simulink model "SR_SNN_Extrinsic_code"  (R2022a)
settings: Solver=FixedStepAuto  StartTime=0.0  StopTime=NTimeSteps  FixedStep=Ts  RelTol=1e-3
values from neighbouring files (symbols this model uses):
  a1 = 5    [SR_Main_Script_Sim.m]
  b = 2    [SR_Main_Script_Sim.m]
  Etol = 10    [SR_Main_Script_Sim.m]
  Mu = 0    [SR_Main_Script_Sim.m]
  NObservations = 10    [SR_Main_Script_Sim.m]
  NStepPerTarget = NTimeSteps/NObservations    (= 1)    [SR_Main_Script_Sim.m]
  r = 0.14*0.5*10    (= 0.7)    [SR_Main_Script_Sim.m]
  s1 = 900    [ConditionCheck.m]    (also in MySNN.m = 0)
  s2 = 900    [ConditionCheck.m]    (also in MySNN.m = 0)
  s3 = 900    [ConditionCheck.m]    (also in MySNN.m = 0)
  Ts = 1e-3    (= 0.001)    [SR_Main_Script_Sim.m]
  Tx = 1    [SR_Main_Script_Sim.m]
  Txi = r*cos(xx)    [SR_Main_Script_Sim.m]
  Ty = 1    [SR_Main_Script_Sim.m]
  Tyi = r*sin(xx)    [SR_Main_Script_Sim.m]
  Tz = 2    [SR_Main_Script_Sim.m]
  v1 = v1 - vMax*(s3/sMin)    [ConditionCheck.m]
  v2 = v2 - vMax*(s3/sMin)    [ConditionCheck.m]
  v3 = v3 - vMax*(s2/sMin)    [ConditionCheck.m]
  v4 = 0    [ConditionCheck.m]
  v5 = 0    [ConditionCheck.m]
  v6 = 0    [ConditionCheck.m]
  v7 = 0    [ConditionCheck.m]
  v8 = 0    [ConditionCheck.m]
  Var = 5    [SR_Main_Script_Sim.m]
  x_i = [[1] ... (first row only)    [SR_Main_Script_Sim.m]
undefined symbols (not defined in the file or in its folder): ConditionCheck, dev_handle, s4, s5, s6, setSup, U1, U2, U3
libraries: slpidlib x4, cstblocks x3
settings Model: SimulationMode=accelerator  Creator=Pouya  LastModifiedBy=Pouya
settings DebuggingCC: UnconnectedInputMsg=warning  UnconnectedOutputMsg=warning  UnconnectedLineMsg=warning
settings RTWCC: DLArmComputeVersion=19.05

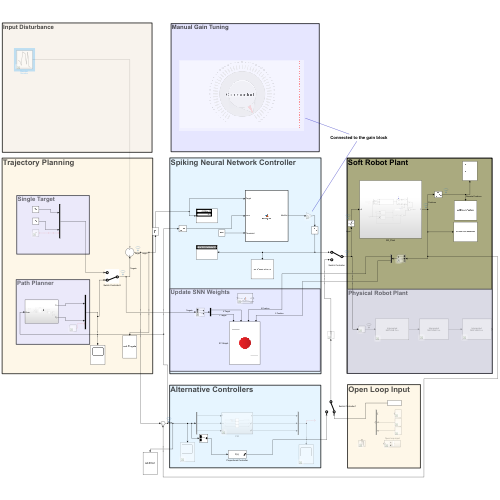
[thumbnail: Simulink's stored preview of the top-level diagram]
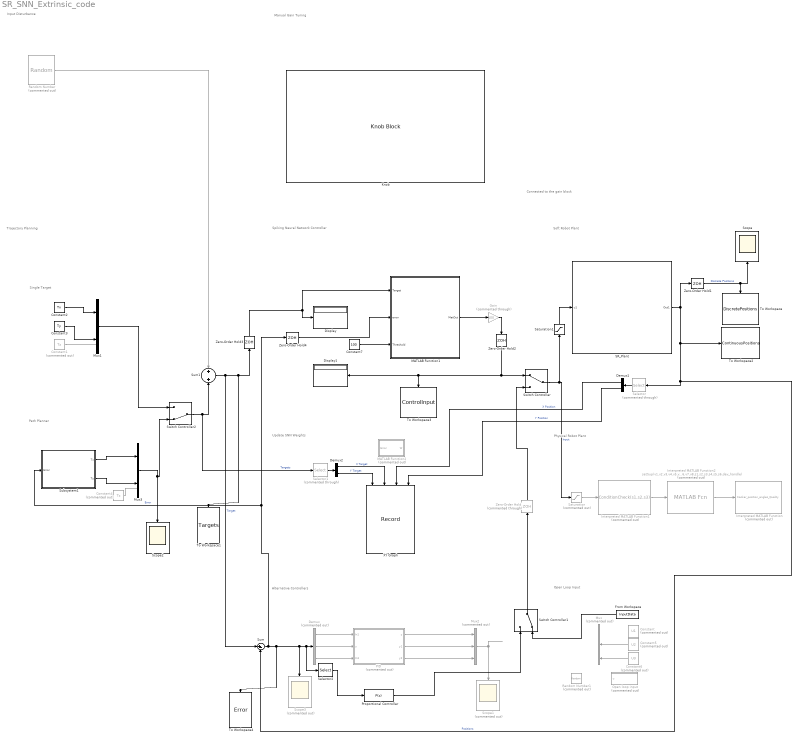
== system SR_SNN_Extrinsic_code ==
  note: Connected to the gain block
  note: Manual Gain Tuning
  note: Physical Robot Plant
  note: Update SNN Weights
  note: Input Disturbance
  note: Path Planner
  note: Single Target
  note: Open Loop Input
  note: Alternative Controllers
  note: Trajectory Planning
  note: Soft Robot Plant
  note: Spiking Neural Network Controller
  Constant : Constant  Commented=on  Value=U1
  Constant1 : Constant  Commented=on  Value=Tz
  Constant2 : Constant  Value=Tx
  Constant3 : Constant  Value=Ty
  Constant4 : Constant  Commented=on  Value=Tz
  Constant5 : Constant  Commented=on  Value=U2
  Constant6 : Constant  Commented=on  Value=U3
  Constant7 : Constant  Value=100
  Demux : Demux  Commented=on  Outputs=3
  Demux1 : Demux  Outputs=2
  Demux2 : Demux  Outputs=2
  Display : Display
  Display1 : Display
  From Workspace : FromWorkspace  VariableName=InputData  SampleTime=Ts
  Gain : Gain  Commented=through  Gain=100
  Interpreted MATLAB Function : MATLABFcn  Commented=on  MATLABFcn=tracker_position_angles_Quality
  Interpreted MATLAB Function1 : MATLABFcn  Commented=on  MATLABFcn=ConditionCheck(s1,s2,s3)
  Interpreted MATLAB Function2 : MATLABFcn  Commented=on  MATLABFcn=setSup(v1,v2,v3,v4,v5,v6,v7,v8,s1,s2,s3,s4,s5,s6,dev_handle)
  Knob : KnobBlock
  MATLAB Function1 : MATLAB Function  TreatAsAtomicUnit=on
  MATLAB Function2 : MATLAB Function  Commented=on  TreatAsAtomicUnit=on
  Mux : Mux  Commented=on  Inputs=3
  Mux1 : Mux  Inputs=2
  Mux2 : Mux  Commented=on  Inputs=3
  Mux3 : Mux  Inputs=2
  Open loop input : Subsystem  Commented=on
  PID : Subsystem  Commented=on
  Proportional Controller : slpidlib/PID Controller  Controller=P  Form=Parallel  TimeDomain=Discrete-time  UseExternalTs=off  SampleTime=-1  IntegratorMethod=Forward Euler  FilterMethod=Forward Euler  ControllerParametersSource=internal  P=150  I=0.1  UseKiTs=off  D=0  N=100  UseFilter=on  TunerSelectOption=Transfer Function Based (PID Tuner App)  InitialConditionSource=internal  InitialConditionForIntegrator=1  InitialConditionForFilter=0  DifferentiatorICPrevScaledInput=0  ExternalReset=none  TrackingMode=off  Kt=1  LimitOutput=on  SatLimitsSource=internal  UpperSaturationLimit=1  LowerSaturationLimit=0  LinearizeAsGain=off  AntiWindupMode=none  Kb=1  POutMin=[]  POutMax=[]  IOutMin=[]  IOutMax=[]  DOutMin=[]  DOutMax=[]  NOutMin=[]  NOutMax=[]  SumOutMin=[]  SumOutMax=[]  SaturationOutMin=[]  SaturationOutMax=[]  PParamMin=[]  PParamMax=[]  IParamMin=[]  IParamMax=[]  DParamMin=[]  DParamMax=[]  NParamMin=[]  NParamMax=[]  KbParamMin=[]  KbParamMax=[]  KtParamMin=[]  KtParamMax=[]  KbOutMin=[]  KbOutMax=[]  KtOutMin=[]  KtOutMax=[]  IntegratorOutMin=[]  IntegratorOutMax=[]  FilterOutMin=[]  FilterOutMax=[]  SumI1OutMin=[]  SumI1OutMax=[]  SumI2OutMin=[]  SumI2OutMax=[]  SumI3OutMin=[]  SumI3OutMax=[]  SumI4OutMin=[]  SumI4OutMax=[]  SumDOutMin=[]  SumDOutMax=[]  DifferentiatorOutMin=[]  DifferentiatorOutMax=[]  FilterDiffOutCoefMin=[]  FilterDiffOutCoefMax=[]  ReciprocalOutMin=[]  ReciprocalOutMax=[]  SumDenOutMin=[]  SumDenOutMax=[]  SumNumOutMin=[]  SumNumOutMax=[]  DivideOutMin=[]  DivideOutMax=[]  UdiffTsProdOutMin=[]  UdiffTsProdOutMax=[]  NTsProdOutMin=[]  NTsProdOutMax=[]  UintegralTsProdOutMin=[]  UintegralTsProdOutMax=[]  UngainTsProdOutMin=[]  UngainTsProdOutMax=[]  IntegratorContinuousStateAttributes=''  IntegratorStateMustResolveToSignalObject=off  IntegratorRTWStateStorageClass=Auto  FilterContinuousStateAttributes=''  FilterStateMustResolveToSignalObject=off  FilterRTWStateStorageClass=Auto  ParallelPVariant=InternalParameters  IdealPVariant=Disabled  IVariant=Disabled  DVariant=Disabled  IntegratorVariant=Disabled  SatVariant=Enabled  AWVariant=Disabled  PCopyVariant=Disabled  TRVariant=Disabled  FdbkBlocksVariant=Forward  IdealPFdbkVariant=Disabled  SatFdbkVariant=Disabled  DerivativeFilterVariant=Disabled  NVariant=Disabled  NCopyVariant=Disabled_SignalSpec  FilterICVariant=Disabled  IntegratorICVariant=Disabled  ExternalResetVariant=Disabled  TRSumVariant=Passthrough  SumFdbkVariant=Disabled  SumVariant=Passthrough_P  TsampFilterVariant=InternalTs  TsampNgainVariant=Passthrough  TsampIntegralVariant=Disabled_SignalSpec  ExternalSaturationOutDataTypeStr=Inherit: Same as second input  aMode=0
  Random Number : RandomNumber  Commented=on  Mean=Mu  Variance=Var  SampleTime=Ts
  Random Number1 : RandomNumber  Commented=on  SampleTime=Ts
  SR_Plant : Subsystem
  Saturation : Saturate  Commented=on  UpperLimit=4  LowerLimit=-4
  Saturation1 : Saturate  UpperLimit=1  LowerLimit=0
  Scope : Scope
  Scope1 : Scope  Commented=on
  Scope2 : Scope
  Scope3 : Scope  Commented=on
  Selector : Selector  Commented=through  InputPortWidth=3  IndexOptions=Index vector (dialog)  Indices=[1 2]  OutputSizes=1
  Selector1 : Selector  Commented=through  InputPortWidth=3  IndexOptions=Index vector (dialog)  Indices=[1 2]  OutputSizes=1
  Selector2 : Selector  InputPortWidth=2  IndexOptions=Index vector (dialog)  Indices=[1]  OutputSizes=1
  Subsystem1 : Subsystem
  Sum : Sum  Inputs=|+-
  Sum1 : Sum
  Switch Controller : ManualSwitch
  Switch Controller1 : ManualSwitch  CurrentSetting=0
  Switch Controller2 : ManualSwitch  CurrentSetting=0
  To Workspace : ToWorkspace  VariableName=DiscretePositions  SaveFormat=Timeseries  SampleTime=-1
  To Workspace1 : ToWorkspace  VariableName=Targets  SaveFormat=Timeseries  SampleTime=-1
  To Workspace2 : ToWorkspace  VariableName=ContinuousPositions  SaveFormat=Timeseries  SampleTime=-1
  To Workspace3 : ToWorkspace  VariableName=ControlInput  SaveFormat=Timeseries  SampleTime=-1
  To Workspace4 : ToWorkspace  VariableName=Error  SaveFormat=Timeseries  SampleTime=-1
  XY Graph : Record  FileSettingsInternal="{\"entries\":[{\"content\":{\"excelSettings\":{\"content\":{},\"type\":\"Streamout.ExcelSettings\"}},\"type\":\"Streamout.FileSettingStorage\",\"uuid\":\"73c5b73b-fab0-4ab5-94d2-4132d8f4e88e\"}],\"packageUris\":[\"http://schema.mathworks.com/mf0/streamout_blocks/R2020a\"],\"version\":\"1.0\"}"  Layout=[1 1]  SignalsInternal="{\"entries\":[{\"content\":{\"signals\":[{\"content\":{\"blockPath\":[\"SR_SNN_Extrinsic_code/XY Graph\"],\"channel\":[],\"dimensions\":[1],\"domain\":\"SR_SNN_Extrinsic_code/XY Graph\",\"lineColor\":\"#0072bd\",\"plots\":[1,2],\"port\":1,\"sid\":[\"\"],\"signalID\":6157,\"signalName\":\"Y Target\"},\"type\":\"RecordBlkView.Signal\",\"uuid\":\"fa4d0461-3b01-48b9-ba2e-6f3d6dd28ef7\"},{\"content\":{\"blockPath\":[\"SR_SNN_Extrinsic_code/XY Graph\"],\"channel\":[],\"dimensions\":[1],\"domain\":\"SR_SNN_Extrinsic_code/XY Graph\",\"lineColor\":\"#0072bd\",\"plots\":[1,2],\"port\":2,\"sid\":[\"\"],\"signalID\":6161,\"signalName\":\"X Target\"},\"type\":\"RecordBlkView.Signal\",\"uuid\":\"838e8c0a-52c2-4c5c-8dac-cd2bc88a20a1\"},{\"content\":{\"blockPath\":[\"SR_SNN_Extrinsic_code/XY Graph\"],\"channel\":[],\"dimensions\":[1],\"domain\":\"SR_SNN_Extrinsic_code/XY Graph\",\"lineColor\":\"#d95319\",\"lineStyle\":\"DOTTED\",\"plots\":[1,2],\"port\":3,\"sid\":[\"\"],\"signalID\":6165,\"signalName\":\"X Position\"},\"type\":\"RecordBlkView.Signal\",\"uuid\":\"8dc49ed9-1307-4fcf-8461-6fcf0d652c4a\"},{\"content\":{\"blockPath\":[\"SR_SNN_Extrinsic_code/XY Graph\"],\"channel\":[],\"dimensions\":[1],\"domain\":\"SR_SNN_Extrinsic_code/XY Graph\",\"lineColor\":\"#d95319\",\"lineStyle\":\"DOTTED\",\"plots\":[1,2],\"port\":4,\"sid\":[\"\"],\"signalID\":6169,\"signalName\":\"Y Position\"},\"type\":\"RecordBlkView.Signal\",\"uuid\":\"e0714d31-97f1-4acd-9cba-ab512efbf2cd\"}]},\"type\":\"RecordBlkView.InputSignals\",\"uuid\":\"e6cc7207-a460-4614-bf63-22bf2ecd2d00\"}],\"packageUris\":[\"http://schema.mathworks.com/mf0/streamout_blocks/R2020a\"],\"version\":\"1.0\"}"  VisualizationBindings="{\"xyplotplugin\":{\"info\":[{\"series\":[{\"bindingParametersList\":[{\"parameter\":\"Y-Axis\",\"signalID\":6157,\"signalName\":\"Y Target\"},{\"parameter\":\"X-Axis\",\"signalID\":6161,\"signalName\":\"X Target\"}],\"seriesID\":9808},{\"bindingParametersList\":[{\"parameter\":\"X-Axis\",\"signalID\":6165,\"signalName\":\"X Position\"},{\"parameter\":\"Y-Axis\",\"signalID\":6169,\"signalName\":\"Y Position\"}],\"seriesID\":48772}],\"subplotID\":1}]}}"  CompatibilityTag=XY
  Zero-Order Hold : ZeroOrderHold  Commented=through  SampleTime=Ts
  Zero-Order Hold{1..4} (4 alike) : ZeroOrderHold  SampleTime=Ts
  wires:
  Constant2/1 -> Mux1/1
  Constant3/1 -> Mux1/2
  SR_Plant/1(Out1) -> Sum/2, Selector/1, To Workspace2/1, Zero-Order Hold1/1  "Positions"
  Constant1/1 -> ?
  Switch Controller1/1 -> Zero-Order Hold/1
  Zero-Order Hold/1 -> Switch Controller/2
  Demux/2 -> PID/2(u)
  Demux/1 -> PID/1(In1)
  Demux/3 -> PID/3(In3)
  PID/1(y) -> Mux2/1
  Switch Controller/1 -> Saturation/1, Saturation1/1  "Input"
  PID/2(y1) -> Mux2/2
  PID/3(y2) -> Mux2/3
  Mux2/1 -> Scope1/1
  Mux1/1 -> Switch Controller2/1
  Mux3/1 -> Switch Controller2/2, Scope2/1
  Subsystem1/2(Ty) -> Mux3/2
  Subsystem1/1(Tx) -> Mux3/1
  Constant4/1 -> ?
  Sum/1 -> Scope3/1, Selector2/1, Demux/1, To Workspace4/1, Zero-Order Hold4/1, Subsystem1/1(Error)  "Error"
  Zero-Order Hold1/1 -> Scope/1, To Workspace/1  "Discrete Positions"
  Random Number/1 -> Sum1/1
  Sum1/1 -> Sum/1, Zero-Order Hold3/1, To Workspace1/1  "Target"
  MATLAB Function1/1(MatOut) -> Gain/1
  Zero-Order Hold3/1 -> MATLAB Function1/1(Target), Display/1
  Zero-Order Hold2/1 -> Switch Controller/1, Display1/1, To Workspace3/1
  Zero-Order Hold4/1 -> MATLAB Function1/2(error)
  Saturation/1 -> Interpreted MATLAB Function1/1
  Interpreted MATLAB Function1/1 -> Interpreted MATLAB Function2/1
  Interpreted MATLAB Function2/1 -> Interpreted MATLAB Function/1
  Gain/1 -> Zero-Order Hold2/1
  Saturation1/1 -> SR_Plant/1(u1)
  Selector/1 -> Demux1/1
  Demux1/1 -> XY Graph/3  "X Position"
  Demux1/2 -> XY Graph/4  "Y Position"
  Selector1/1 -> Demux2/1
  Switch Controller2/1 -> Selector1/1, Sum1/2  "Targets"
  Demux2/2 -> XY Graph/1  "Y Target"
  Demux2/1 -> XY Graph/2  "X Target"
  Constant5/1 -> Mux/2
  Constant6/1 -> Mux/3
  From Workspace/1 -> Switch Controller1/2
  Constant7/1 -> MATLAB Function1/3(Threshold)
  Proportional Controller/1 -> Switch Controller1/1
  Selector2/1 -> Proportional Controller/1

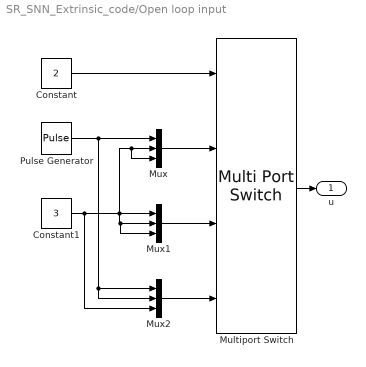
== system SR_SNN_Extrinsic_code/Open loop input ==
  Constant : Constant  Value=2
  Constant1 : Constant  Value=3
  Multiport Switch : MultiPortSwitch  SaturateOnIntegerOverflow=off  InputSameDT=off
  Mux : Mux  Inputs=3
  Mux1 : Mux  Inputs=3
  Mux2 : Mux  Inputs=3
  Pulse Generator : DiscretePulseGenerator  PulseType=Time based  Period=5  PulseWidth=10
  u : Outport
  wires:
  Constant1/1 -> Mux2/3, Mux1/3, Mux1/2, Mux1/1, Mux/3, Mux/2
  Pulse Generator/1 -> Mux2/2, Mux2/1, Mux/1
  Constant/1 -> Multiport Switch/1
  Mux2/1 -> Multiport Switch/4
  Mux/1 -> Multiport Switch/2
  Multiport Switch/1 -> u/1
  Mux1/1 -> Multiport Switch/3

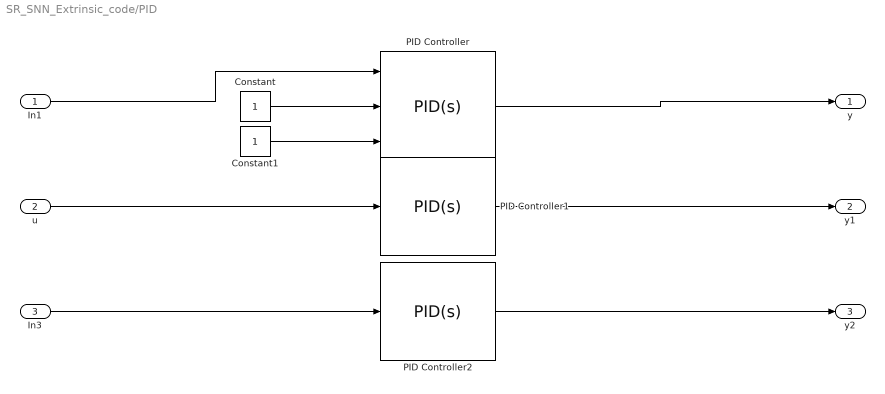
== system SR_SNN_Extrinsic_code/PID ==
  In1 : Inport
  u : Inport  Port=2
  In3 : Inport  Port=3
  Constant : Constant
  Constant1 : Constant
  PID Controller : slpidlib/PID Controller  Controller=PID  Form=Parallel  TimeDomain=Continuous-time  UseExternalTs=off  SampleTime=-1  IntegratorMethod=Forward Euler  FilterMethod=Forward Euler  ControllerParametersSource=internal  P=-18.4443035779301  I=-965.50333327494  UseKiTs=off  D=0.00626834007376685  N=2942.45420013505  UseFilter=on  TunerSelectOption=Transfer Function Based (PID Tuner App)  InitialConditionSource=external  InitialConditionForIntegrator=0  InitialConditionForFilter=0  DifferentiatorICPrevScaledInput=0  ExternalReset=none  TrackingMode=off  Kt=1  LimitOutput=off  SatLimitsSource=internal  UpperSaturationLimit=inf  LowerSaturationLimit=-inf  LinearizeAsGain=on  AntiWindupMode=none  Kb=1  POutMin=[]  POutMax=[]  IOutMin=[]  IOutMax=[]  DOutMin=[]  DOutMax=[]  NOutMin=[]  NOutMax=[]  SumOutMin=[]  SumOutMax=[]  SaturationOutMin=[]  SaturationOutMax=[]  PParamMin=[]  PParamMax=[]  IParamMin=[]  IParamMax=[]  DParamMin=[]  DParamMax=[]  NParamMin=[]  NParamMax=[]  KbParamMin=[]  KbParamMax=[]  KtParamMin=[]  KtParamMax=[]  KbOutMin=[]  KbOutMax=[]  KtOutMin=[]  KtOutMax=[]  IntegratorOutMin=[]  IntegratorOutMax=[]  FilterOutMin=[]  FilterOutMax=[]  SumI1OutMin=[]  SumI1OutMax=[]  SumI2OutMin=[]  SumI2OutMax=[]  SumI3OutMin=[]  SumI3OutMax=[]  SumI4OutMin=[]  SumI4OutMax=[]  SumDOutMin=[]  SumDOutMax=[]  DifferentiatorOutMin=[]  DifferentiatorOutMax=[]  FilterDiffOutCoefMin=[]  FilterDiffOutCoefMax=[]  ReciprocalOutMin=[]  ReciprocalOutMax=[]  SumDenOutMin=[]  SumDenOutMax=[]  SumNumOutMin=[]  SumNumOutMax=[]  DivideOutMin=[]  DivideOutMax=[]  UdiffTsProdOutMin=[]  UdiffTsProdOutMax=[]  NTsProdOutMin=[]  NTsProdOutMax=[]  UintegralTsProdOutMin=[]  UintegralTsProdOutMax=[]  UngainTsProdOutMin=[]  UngainTsProdOutMax=[]  IntegratorContinuousStateAttributes=''  IntegratorStateMustResolveToSignalObject=off  IntegratorRTWStateStorageClass=Auto  FilterContinuousStateAttributes=''  FilterStateMustResolveToSignalObject=off  FilterRTWStateStorageClass=Auto  ParallelPVariant=InternalParameters  IdealPVariant=Disabled  IVariant=InternalParameters  DVariant=InternalParameters  IntegratorVariant=Continuous  SatVariant=Disabled  AWVariant=Passthrough  PCopyVariant=Disabled  TRVariant=Disabled  FdbkBlocksVariant=Forward  IdealPFdbkVariant=Disabled  SatFdbkVariant=Disabled  DerivativeFilterVariant=ContFilter  NVariant=InternalParameters  NCopyVariant=Disabled  FilterICVariant=ExternalICs  IntegratorICVariant=ExternalICs  ExternalResetVariant=Disabled  TRSumVariant=Passthrough  SumFdbkVariant=Disabled  SumVariant=Sum_PID  TsampFilterVariant=InternalTs  TsampNgainVariant=Passthrough  TsampIntegralVariant=Passthrough  ExternalSaturationOutDataTypeStr=Inherit: Same as second input  aMode=0
  PID Controller1 : slpidlib/PID Controller  Controller=PID  Form=Parallel  TimeDomain=Continuous-time  UseExternalTs=off  SampleTime=-1  IntegratorMethod=Forward Euler  FilterMethod=Forward Euler  ControllerParametersSource=internal  P=0.79056648520257  I=12.0335076656055  UseKiTs=off  D=0.00902589117456867  N=93.9877255340492  UseFilter=on  TunerSelectOption=Transfer Function Based (PID Tuner App)  InitialConditionSource=internal  InitialConditionForIntegrator=0  InitialConditionForFilter=0  DifferentiatorICPrevScaledInput=0  ExternalReset=none  TrackingMode=off  Kt=1  LimitOutput=off  SatLimitsSource=internal  UpperSaturationLimit=inf  LowerSaturationLimit=-inf  LinearizeAsGain=on  AntiWindupMode=none  Kb=1  POutMin=[]  POutMax=[]  IOutMin=[]  IOutMax=[]  DOutMin=[]  DOutMax=[]  NOutMin=[]  NOutMax=[]  SumOutMin=[]  SumOutMax=[]  SaturationOutMin=[]  SaturationOutMax=[]  PParamMin=[]  PParamMax=[]  IParamMin=[]  IParamMax=[]  DParamMin=[]  DParamMax=[]  NParamMin=[]  NParamMax=[]  KbParamMin=[]  KbParamMax=[]  KtParamMin=[]  KtParamMax=[]  KbOutMin=[]  KbOutMax=[]  KtOutMin=[]  KtOutMax=[]  IntegratorOutMin=[]  IntegratorOutMax=[]  FilterOutMin=[]  FilterOutMax=[]  SumI1OutMin=[]  SumI1OutMax=[]  SumI2OutMin=[]  SumI2OutMax=[]  SumI3OutMin=[]  SumI3OutMax=[]  SumI4OutMin=[]  SumI4OutMax=[]  SumDOutMin=[]  SumDOutMax=[]  DifferentiatorOutMin=[]  DifferentiatorOutMax=[]  FilterDiffOutCoefMin=[]  FilterDiffOutCoefMax=[]  ReciprocalOutMin=[]  ReciprocalOutMax=[]  SumDenOutMin=[]  SumDenOutMax=[]  SumNumOutMin=[]  SumNumOutMax=[]  DivideOutMin=[]  DivideOutMax=[]  UdiffTsProdOutMin=[]  UdiffTsProdOutMax=[]  NTsProdOutMin=[]  NTsProdOutMax=[]  UintegralTsProdOutMin=[]  UintegralTsProdOutMax=[]  UngainTsProdOutMin=[]  UngainTsProdOutMax=[]  IntegratorContinuousStateAttributes=''  IntegratorStateMustResolveToSignalObject=off  IntegratorRTWStateStorageClass=Auto  FilterContinuousStateAttributes=''  FilterStateMustResolveToSignalObject=off  FilterRTWStateStorageClass=Auto  ParallelPVariant=InternalParameters  IdealPVariant=Disabled  IVariant=InternalParameters  DVariant=InternalParameters  IntegratorVariant=Continuous  SatVariant=Disabled  AWVariant=Passthrough  PCopyVariant=Disabled  TRVariant=Disabled  FdbkBlocksVariant=Forward  IdealPFdbkVariant=Disabled  SatFdbkVariant=Disabled  DerivativeFilterVariant=ContFilter  NVariant=InternalParameters  NCopyVariant=Disabled  FilterICVariant=InternalICsFilter  IntegratorICVariant=InternalICs  ExternalResetVariant=Disabled  TRSumVariant=Passthrough  SumFdbkVariant=Disabled  SumVariant=Sum_PID  TsampFilterVariant=InternalTs  TsampNgainVariant=Passthrough  TsampIntegralVariant=Passthrough  ExternalSaturationOutDataTypeStr=Inherit: Same as second input  aMode=0
  PID Controller2 : slpidlib/PID Controller  Controller=PID  Form=Parallel  TimeDomain=Continuous-time  UseExternalTs=off  SampleTime=-1  IntegratorMethod=Forward Euler  FilterMethod=Forward Euler  ControllerParametersSource=internal  P=0.559243071667532  I=12.7287987560963  UseKiTs=off  D=0  N=100  UseFilter=on  TunerSelectOption=Transfer Function Based (PID Tuner App)  InitialConditionSource=internal  InitialConditionForIntegrator=0  InitialConditionForFilter=0  DifferentiatorICPrevScaledInput=0  ExternalReset=none  TrackingMode=off  Kt=1  LimitOutput=off  SatLimitsSource=internal  UpperSaturationLimit=inf  LowerSaturationLimit=-inf  LinearizeAsGain=on  AntiWindupMode=none  Kb=1  POutMin=[]  POutMax=[]  IOutMin=[]  IOutMax=[]  DOutMin=[]  DOutMax=[]  NOutMin=[]  NOutMax=[]  SumOutMin=[]  SumOutMax=[]  SaturationOutMin=[]  SaturationOutMax=[]  PParamMin=[]  PParamMax=[]  IParamMin=[]  IParamMax=[]  DParamMin=[]  DParamMax=[]  NParamMin=[]  NParamMax=[]  KbParamMin=[]  KbParamMax=[]  KtParamMin=[]  KtParamMax=[]  KbOutMin=[]  KbOutMax=[]  KtOutMin=[]  KtOutMax=[]  IntegratorOutMin=[]  IntegratorOutMax=[]  FilterOutMin=[]  FilterOutMax=[]  SumI1OutMin=[]  SumI1OutMax=[]  SumI2OutMin=[]  SumI2OutMax=[]  SumI3OutMin=[]  SumI3OutMax=[]  SumI4OutMin=[]  SumI4OutMax=[]  SumDOutMin=[]  SumDOutMax=[]  DifferentiatorOutMin=[]  DifferentiatorOutMax=[]  FilterDiffOutCoefMin=[]  FilterDiffOutCoefMax=[]  ReciprocalOutMin=[]  ReciprocalOutMax=[]  SumDenOutMin=[]  SumDenOutMax=[]  SumNumOutMin=[]  SumNumOutMax=[]  DivideOutMin=[]  DivideOutMax=[]  UdiffTsProdOutMin=[]  UdiffTsProdOutMax=[]  NTsProdOutMin=[]  NTsProdOutMax=[]  UintegralTsProdOutMin=[]  UintegralTsProdOutMax=[]  UngainTsProdOutMin=[]  UngainTsProdOutMax=[]  IntegratorContinuousStateAttributes=''  IntegratorStateMustResolveToSignalObject=off  IntegratorRTWStateStorageClass=Auto  FilterContinuousStateAttributes=''  FilterStateMustResolveToSignalObject=off  FilterRTWStateStorageClass=Auto  ParallelPVariant=InternalParameters  IdealPVariant=Disabled  IVariant=InternalParameters  DVariant=InternalParameters  IntegratorVariant=Continuous  SatVariant=Disabled  AWVariant=Passthrough  PCopyVariant=Disabled  TRVariant=Disabled  FdbkBlocksVariant=Forward  IdealPFdbkVariant=Disabled  SatFdbkVariant=Disabled  DerivativeFilterVariant=ContFilter  NVariant=InternalParameters  NCopyVariant=Disabled  FilterICVariant=InternalICsFilter  IntegratorICVariant=InternalICs  ExternalResetVariant=Disabled  TRSumVariant=Passthrough  SumFdbkVariant=Disabled  SumVariant=Sum_PID  TsampFilterVariant=InternalTs  TsampNgainVariant=Passthrough  TsampIntegralVariant=Passthrough  ExternalSaturationOutDataTypeStr=Inherit: Same as second input  aMode=0
  y : Outport
  y1 : Outport  Port=2
  y2 : Outport  Port=3
  wires:
  u/1 -> PID Controller1/1
  PID Controller/1 -> y/1
  In1/1 -> PID Controller/1
  PID Controller1/1 -> y1/1
  In3/1 -> PID Controller2/1
  PID Controller2/1 -> y2/1
  Constant/1 -> PID Controller/2
  Constant1/1 -> PID Controller/3

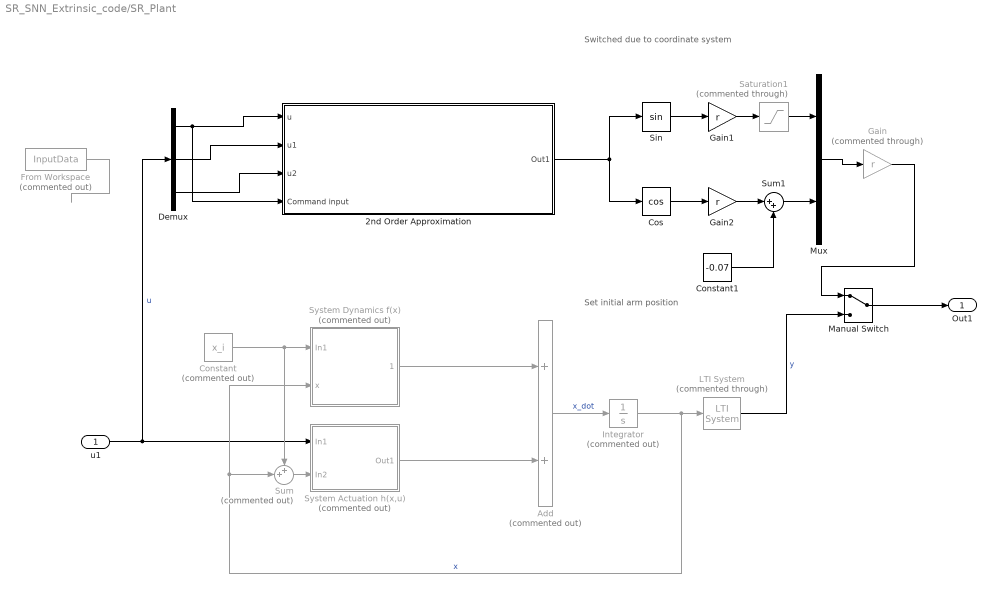
== system SR_SNN_Extrinsic_code/SR_Plant ==
  note: Set initial arm position
  note: Switched due to coordinate system
  u1 : Inport
  2nd Order Approximation : Subsystem
  Add : Sum  Commented=on
  Constant : Constant  Commented=on  Value=x_i
  Constant1 : Constant  Value=-0.07
  Cos : Trigonometry  Operator=cos
  Demux : Demux  Outputs=3
  From Workspace : FromWorkspace  Commented=on  VariableName=InputData
  Gain : Gain  Commented=through  Gain=r
  Gain1 : Gain  Gain=r
  Gain2 : Gain  Gain=r
  Integrator : Integrator  Commented=on
  LTI System : cstblocks/LTI System  Commented=through  sys=C  IC=[]
  Manual Switch : ManualSwitch
  Mux : Mux  Inputs=2
  Saturation1 : Saturate  Commented=through  UpperLimit=r  LowerLimit=0
  Sin : Trigonometry
  Sum : Sum  Commented=on  Inputs=++|
  Sum1 : Sum  Inputs=|++
  System Actuation h(x,u) : Subsystem  Commented=on
  System Dynamics f(x) : Subsystem  Commented=on
  Out1 : Outport
  wires:
  u1/1 -> Demux/1, System Actuation h(x,u)/1(In1)  "u"
  System Dynamics f(x)/1(1) -> Add/1
  System Actuation h(x,u)/1(Out1) -> Add/2
  Add/1 -> Integrator/1  "x_dot"
  Constant/1 -> Sum/1, System Dynamics f(x)/1(In1)
  Integrator/1 -> System Dynamics f(x)/2(x), Sum/2, LTI System/1  "x"
  LTI System/1 -> Manual Switch/2  "y"
  Sum/1 -> System Actuation h(x,u)/2(In2)
  2nd Order Approximation/1(Out1) -> Cos/1, Sin/1
  Manual Switch/1 -> Out1/1
  Demux/1 -> 2nd Order Approximation/4(Command input), 2nd Order Approximation/1(u)
  Demux/2 -> 2nd Order Approximation/2(u1)
  Demux/3 -> 2nd Order Approximation/3(u2)
  From Workspace/1 -> ?
  Sin/1 -> Gain1/1
  Cos/1 -> Gain2/1
  Gain/1 -> Manual Switch/1
  Gain2/1 -> Sum1/1
  Gain1/1 -> Saturation1/1
  Sum1/1 -> Mux/2
  Saturation1/1 -> Mux/1
  Mux/1 -> Gain/1
  Constant1/1 -> Sum1/2

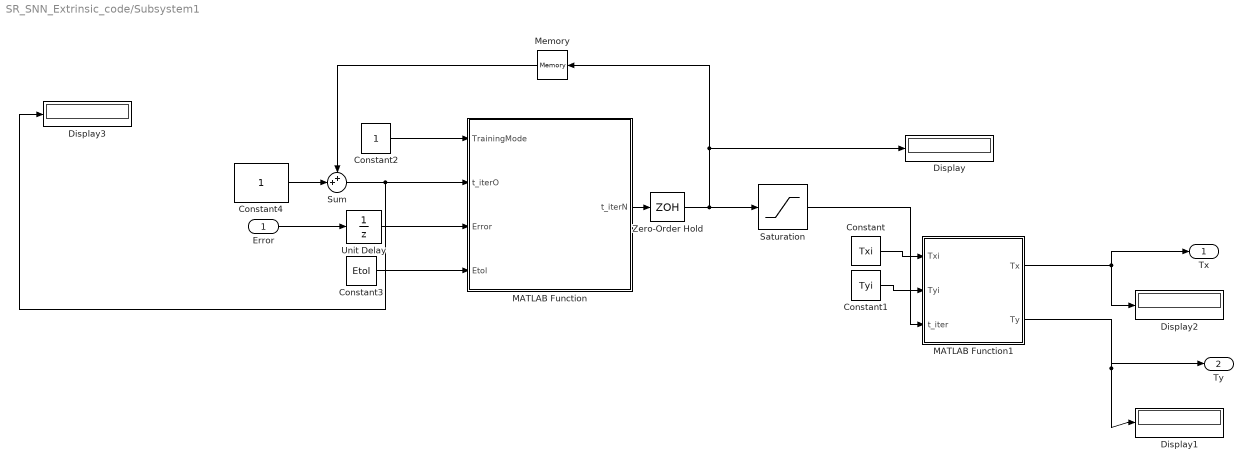
== system SR_SNN_Extrinsic_code/Subsystem1 ==
  Error : Inport
  Constant : Constant  Value=Txi
  Constant1 : Constant  Value=Tyi
  Constant2 : Constant
  Constant3 : Constant  Value=Etol
  Constant4 : Constant
  Display{,1..3} (4 alike) : Display
  MATLAB Function : MATLAB Function  TreatAsAtomicUnit=on
  MATLAB Function1 : MATLAB Function  TreatAsAtomicUnit=on
  Memory : Memory  InheritSampleTime=on  LinearizeAsDelay=on
  Saturation : Saturate  UpperLimit=NObservations  LowerLimit=0
  Sum : Sum  Inputs=++|
  Unit Delay : UnitDelay  SampleTime=-1  HasFrameUpgradeWarning=on
  Zero-Order Hold : ZeroOrderHold  SampleTime=NStepPerTarget
  Tx : Outport
  Ty : Outport  Port=2
  wires:
  MATLAB Function1/1(Tx) -> Tx/1, Display2/1
  MATLAB Function1/2(Ty) -> Display1/1, Ty/1
  Error/1 -> Unit Delay/1
  Constant3/1 -> MATLAB Function/4(Etol)
  MATLAB Function/1(t_iterN) -> Zero-Order Hold/1
  Unit Delay/1 -> MATLAB Function/3(Error)
  Constant4/1 -> Sum/2
  Constant1/1 -> MATLAB Function1/2(Tyi)
  Constant/1 -> MATLAB Function1/1(Txi)
  Constant2/1 -> MATLAB Function/1(TrainingMode)
  Memory/1 -> Sum/1
  Saturation/1 -> MATLAB Function1/3(t_iter)
  Zero-Order Hold/1 -> Display/1, Memory/1, Saturation/1
  Sum/1 -> MATLAB Function/2(t_iterO), Display3/1

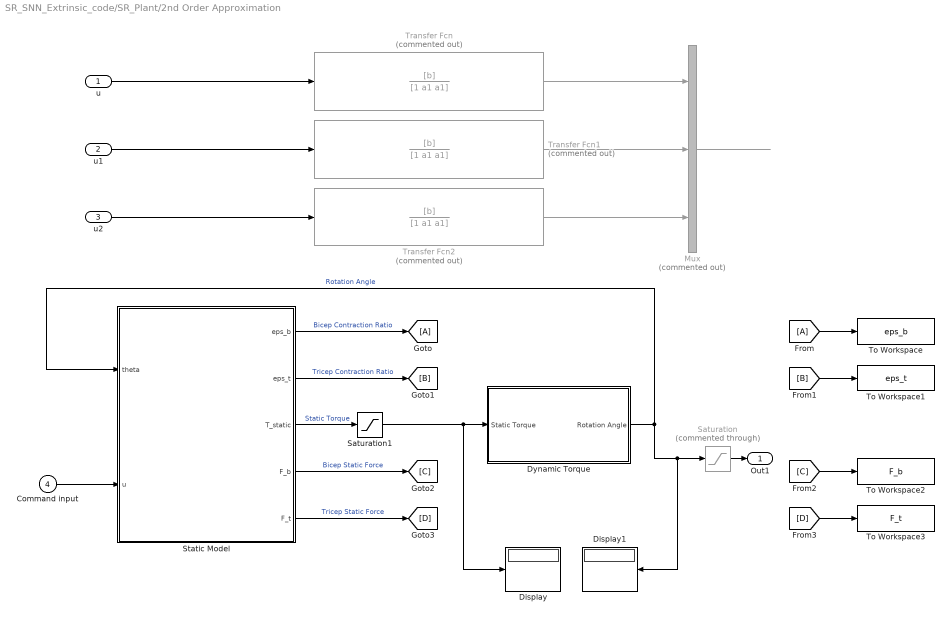
== system SR_SNN_Extrinsic_code/SR_Plant/2nd Order Approximation ==
  u : Inport
  u1 : Inport  Port=2
  u2 : Inport  Port=3
  Command input : Inport  Port=4
  Display : Display
  Display1 : Display
  Dynamic Torque : Subsystem
  From : From
  Goto : Goto
  Mux : Mux  Commented=on  Inputs=3
  Saturation : Saturate  Commented=through  UpperLimit=pi  LowerLimit=-pi
  Saturation1 : Saturate  UpperLimit=35  LowerLimit=-35
  Static Model : MATLAB Function  TreatAsAtomicUnit=on
  To Workspace : ToWorkspace  VariableName=eps_b  SaveFormat=Timeseries  SampleTime=-1
  To Workspace1 : ToWorkspace  VariableName=eps_t  SaveFormat=Timeseries  SampleTime=-1
  To Workspace2 : ToWorkspace  VariableName=F_b  SaveFormat=Timeseries  SampleTime=-1
  To Workspace3 : ToWorkspace  VariableName=F_t  SaveFormat=Timeseries  SampleTime=-1
  Transfer Fcn : TransferFcn  Commented=on  Numerator=[b]  Denominator=[1 a1 a1]
  Transfer Fcn1 : TransferFcn  Commented=on  Numerator=[b]  Denominator=[1 a1 a1]
  Transfer Fcn2 : TransferFcn  Commented=on  Numerator=[b]  Denominator=[1 a1 a1]
  Out1 : Outport
  wires:
  Transfer Fcn/1 -> Mux/1
  u/1 -> Transfer Fcn/1
  Transfer Fcn1/1 -> Mux/2
  Transfer Fcn2/1 -> Mux/3
  Mux/1 -> ?
  u2/1 -> Transfer Fcn2/1
  u1/1 -> Transfer Fcn1/1
  Command input/1 -> Static Model/2(u)
  From/1 -> To Workspace/1
  [C] -> To Workspace2/1
  Static Model/5(F_t) -> [D]  "Tricep Static Force"
  [B] -> To Workspace1/1
  [D] -> To Workspace3/1
  Static Model/1(eps_b) -> Goto/1  "Bicep Contraction Ratio"
  Dynamic Torque/1(Rotation Angle) -> Static Model/1(theta), Display1/1, Saturation/1  "Rotation Angle"
  Static Model/3(T_static) -> Saturation1/1  "Static Torque"
  Static Model/4(F_b) -> [C]  "Bicep Static Force"
  Static Model/2(eps_t) -> [B]  "Tricep Contraction Ratio"
  Saturation/1 -> Out1/1
  Saturation1/1 -> Display/1, Dynamic Torque/1(Static Torque)

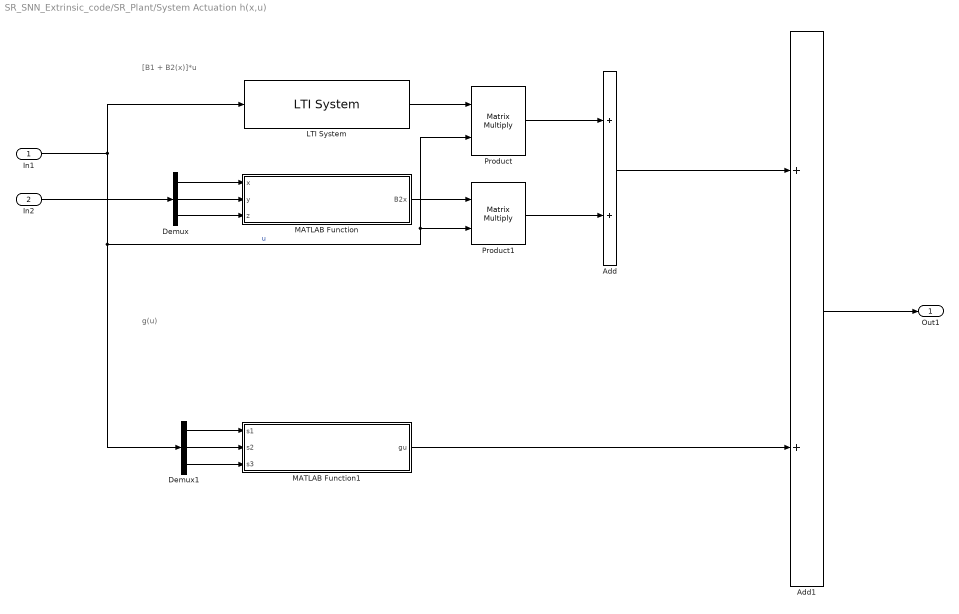
== system SR_SNN_Extrinsic_code/SR_Plant/System Actuation h(x,u) ==
  note: g(u)
  note: [B1 + B2(x)]*u
  In1 : Inport
  In2 : Inport  Port=2
  Add : Sum
  Add1 : Sum
  Demux : Demux  Outputs=3
  Demux1 : Demux  Outputs=3
  LTI System : cstblocks/LTI System  sys=B1  IC=[]
  MATLAB Function : MATLAB Function  TreatAsAtomicUnit=on
  MATLAB Function1 : MATLAB Function  TreatAsAtomicUnit=on
  Product : Product  Multiplication=Matrix(*)
  Product1 : Product  Multiplication=Matrix(*)
  Out1 : Outport
  wires:
  In1/1 -> LTI System/1, Product/2, Product1/2, Demux1/1  "u"
  MATLAB Function1/1(gu) -> Add1/2
  LTI System/1 -> Product/1
  Product/1 -> Add/1
  Add/1 -> Add1/1
  MATLAB Function/1(B2x) -> Product1/1
  Add1/1 -> Out1/1
  In2/1 -> Demux/1
  Demux/2 -> MATLAB Function/2(y)
  Demux/1 -> MATLAB Function/1(x)
  Demux/3 -> MATLAB Function/3(z)
  Demux1/2 -> MATLAB Function1/2(s2)
  Demux1/1 -> MATLAB Function1/1(s1)
  Demux1/3 -> MATLAB Function1/3(s3)
  Product1/1 -> Add/2

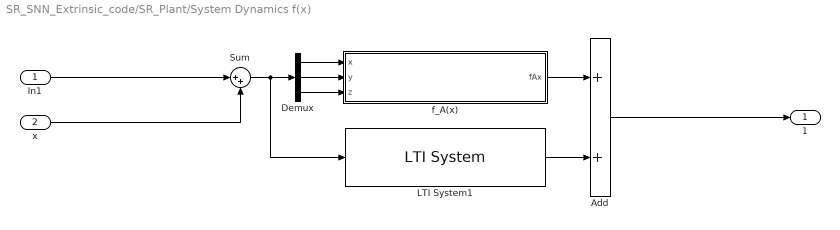
== system SR_SNN_Extrinsic_code/SR_Plant/System Dynamics f(x) ==
  In1 : Inport
  x : Inport  Port=2
  Add : Sum
  Demux : Demux  Outputs=3
  LTI System1 : cstblocks/LTI System  sys=A  IC=[]
  Sum : Sum  Inputs=|++
  f_A(x) : MATLAB Function  TreatAsAtomicUnit=on
  1 : Outport
  wires:
  In1/1 -> Sum/1
  Sum/1 -> LTI System1/1, Demux/1
  Add/1 -> 1/1
  LTI System1/1 -> Add/2
  f_A(x)/1(fAx) -> Add/1
  Demux/1 -> f_A(x)/1(x)
  Demux/2 -> f_A(x)/2(y)
  Demux/3 -> f_A(x)/3(z)
  x/1 -> Sum/2

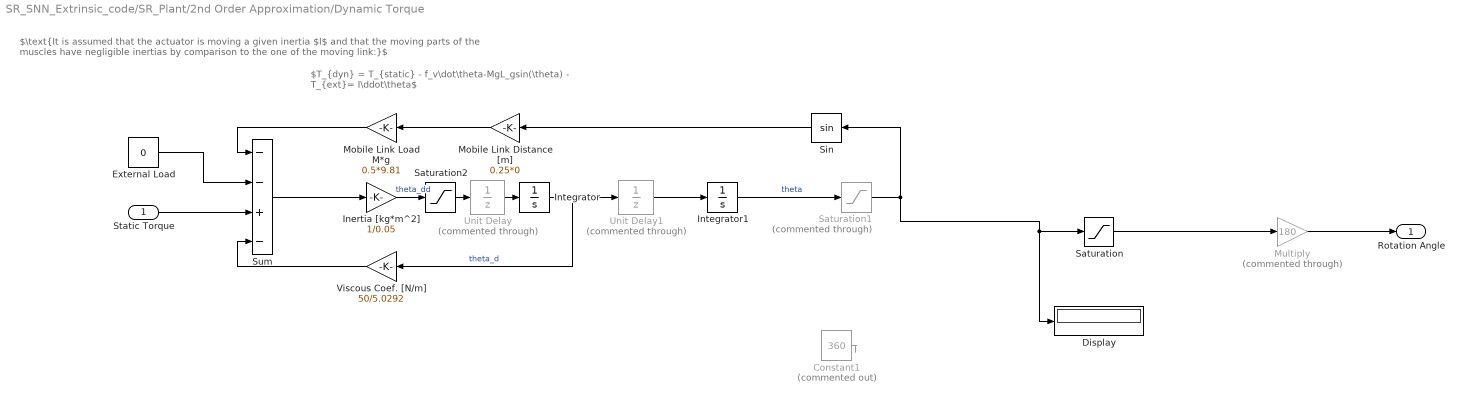
== system SR_SNN_Extrinsic_code/SR_Plant/2nd Order Approximation/Dynamic Torque ==
  note: $T_{dyn} = T_{static} - f_v\dot\theta-MgL_gsin(\theta) - T_{ext}= I\ddot\theta$
  note: $\text{It is assumed that the actuator is moving a given inertia $I$ and that the moving parts of the muscles have negligible inertias by comparison to the one of the moving link:}$
  Static Torque : Inport
  Constant1 : Constant  Commented=on  Value=360
  Display : Display
  External Load : Constant  Value=0
  Inertia [kg*m^2] : Gain  Gain=1/0.05
  Integrator : Integrator
  Integrator1 : Integrator  InitialCondition=1*pi/180
  Mobile Link Distance [m] : Gain  Gain=0.25*0
  Mobile Link Load M*g : Gain  Gain=0.5*9.81
  Multiply : Gain  Commented=through  Gain=180
  Saturation : Saturate  UpperLimit=pi  LowerLimit=0
  Saturation1 : Saturate  Commented=through  UpperLimit=90  LowerLimit=-90
  Saturation2 : Saturate
  Sin : Trigonometry
  Sum : Sum  Inputs=--+-
  Unit Delay : UnitDelay  Commented=through  SampleTime=-1  HasFrameUpgradeWarning=on
  Unit Delay1 : UnitDelay  Commented=through  SampleTime=-1  HasFrameUpgradeWarning=on
  Viscous Coef. [N/m] : Gain  Gain=50/5.0292
  Rotation Angle : Outport
  wires:
  Sum/1 -> Inertia [kg*m^2]/1
  Inertia [kg*m^2]/1 -> Saturation2/1  "theta_dd"
  Integrator/1 -> Viscous Coef. [N/m]/1, Unit Delay1/1  "theta_d"
  Sin/1 -> Mobile Link Distance [m]/1
  Mobile Link Distance [m]/1 -> Mobile Link Load M*g/1
  Static Torque/1 -> Sum/3
  Viscous Coef. [N/m]/1 -> Sum/4
  External Load/1 -> Sum/2
  Mobile Link Load M*g/1 -> Sum/1
  Unit Delay/1 -> Integrator/1
  Unit Delay1/1 -> Integrator1/1
  Integrator1/1 -> Saturation1/1  "theta"
  Constant1/1 -> ?
  Saturation1/1 -> Saturation/1, Display/1, Sin/1
  Saturation/1 -> Multiply/1
  Multiply/1 -> Rotation Angle/1
  Saturation2/1 -> Unit Delay/1

== matlab function SR_SNN_Extrinsic_code/MATLAB Function1 ==
  data: MatOut output; Target input; error input; Threshold input
 function MatOut = RunPython(Target,error,Threshold)
%     MatOut = zeros(3,1);
    MatOut = 0;
    s1=0;s2=0;s3=0;% Has to be preassigned, otherwise Simulink throws an error
    coder.extrinsic('MySNN') % Python functions have to be run extrinsically, meaning no C code generated

    MatOut = MySNN(Target,error,Threshold)
%     [model,s1,s2,s3] = py.SNN_model.Run_model(Target);
    
end

== matlab function SR_SNN_Extrinsic_code/SR_Plant/System Dynamics f(x)/f_A(x) ==
  data: x input; fAx output; y input; z input
function fAx = f_A(x,y,z)

fAx = 10e-3*[[0.17*x^2 - 1.22*y^2 - 0.145*z^2 + 4.92*x*y + 20.3*x*z + 0.748*y*z]
           [3.39*x^2 - 1.94*y^2 + 3.48*z^2 - 1.68*x*y + 5.63*x*z + 17.0*y*z]
           [0.456*x^2 + 0.672*y^2 + 19.4*z^2 - 1.92*x*y + 1.3*x*z - 0.0985*y*z]];

== matlab function SR_SNN_Extrinsic_code/SR_Plant/System Actuation h(x,u)/MATLAB Function ==
  data: x input; B2x output; y input; z input
function B2x = B2(x,y,z)

B2x = 10e-3*[[-2.86*x + 2.34*y + 16.8*z, -2.56*x - 1.23*y - 20.2*z, 1.59*x - 1.16*y + 3.61*z]
             [2.76*x + 0.356*y - 9.28*z, -2.98*x + 3.22*y - 12.9*z, -0.129*x - 4.02*y + 19.9*z]
             [-4.72*x + 3.42*y + 2.26*z, 5.47*x + 3.28*y + 1.58*z, -1.06*x - 6.62*y + 4.49*z]];

== matlab function SR_SNN_Extrinsic_code/SR_Plant/System Actuation h(x,u)/MATLAB Function1 ==
  data: s1 input; gu output; s2 input; s3 input
function gu = g(s1,s2,s3)

gu = 10e-4*[[14.1*s1^2 - 8.48*s2^2 + 5.9*s3^2 - 5.02*s1*s2 - 6.56*s1*s3 + 3.04*s2*s3]
            [11.3*s1^2 - 4.67*s2^2 + 19.5*s3^2 + 1.54*s1*s2 + 3.15*s1*s3 - 1.25*s2*s3]
            [1.05*s1^2 + 2.26*s2^2 + 2.83*s3^2 - 10.6*s1*s2 - 3.2*s1*s3 - 12.7*s2*s3]];

== matlab function SR_SNN_Extrinsic_code/SR_Plant/2nd Order Approximation/Static Model ==
  data: eps_b output; eps_t output; T_static output; F_b output; F_t output; theta input; u input
function [eps_b, eps_t, T_static, F_b, F_t] = fun(theta, u)

F_max = 1000;  % Maximum force of 1000 N
eps_max = 0.25;  % Maximum contraction ratio
a = 0.5;  % Bicep (1) active initial length of 50 cm
b = 0.14*a;
l0 = a;
r = 0.025;

L = sqrt(a^2 + b^2 + 2*a*b*cos(theta));  % AB distance
d = a*b*sin(theta)/L;  % E-AB distance
DL = a + b - L;  % Contracted bicep length variation, DL = L0 - L(theta)
                 % Triceps elongation is r*theta since r is constant

% Actuator (force) static model F(u, eps) = u*F_max*(1 - eps/eps_max) 
% u, normalized control variable in (0, 1)
% eps, contraction ratio of the muscle (L0 - L(theta))/L0 in (0, eps_max)

% => Such a model captures the fundamental variable stiffness spring nature of the
%    skeletal muscle without however being able to take into account the passive tension
%    peculiar to the skeletal muscle.

% => Because the considered muscles are supposed to have the same initial length L0, the
%    following static force model results for biceps and triceps:
eps_b = min(DL/l0, eps_max);
eps_t = max(eps_max - r*theta/l0, 0);

F_b = min(u*F_max*(1 - eps_b/eps_max), F_max);
F_t = min((1 - u)*F_max*(1 - eps_t/eps_max), F_max);

T_static = d*F_b - r*F_t;  % Equilibium torque

% Or, equivalently:
% f = F_max*(d*(1 - DL/(l0*eps_max)) + r^2*theta/(l0*eps_max));
% g = -F_max*r^2*theta/(l0*eps_max);
% 
% T_static = u*f + g;

end

== matlab function SR_SNN_Extrinsic_code/Subsystem1/MATLAB Function ==
  data: TrainingMode input; t_iterO input; Error input; t_iterN output; Etol input
function t_iterN = Target_hit(TrainingMode,t_iterO,Error,Etol)

if TrainingMode == 1
    t_iterN = t_iterO;
    

% else norm(Error) < Etol
%     t_iterN = t_iterO+1;
%     t_iterO = t_iterN;

else
    t_iterN = t_iterO;
end
end

== matlab function SR_SNN_Extrinsic_code/Subsystem1/MATLAB Function1 ==
  data: Txi input; Tx output; Tyi input; t_iter input; Ty output
function [Tx,Ty] = TargetSelector(Txi,Tyi,t_iter)

Tx = Txi(t_iter);
Ty = Tyi(t_iter);

end

== matlab function SR_SNN_Extrinsic_code/MATLAB Function2 ==
  data: Error input; W output
function W = UpdateSNNWeights(Error)
  W=0;% Has to be preassigned, otherwise Simulink throws an error
  coder.extrinsic('py.SNN_model') % Python functions have to be run extrinsically, meaning no C code generated
  W = py.SNN_model.Update(Error);
